simulink model "gm_db2_level5_final_hdlsss"  (R2021a)
settings: Solver=FixedStepDiscrete  StartTime=0.0  StopTime=0.2  RelTol=1e-3
libraries: hdlmdlgenlib x56
(part 2 of 4)

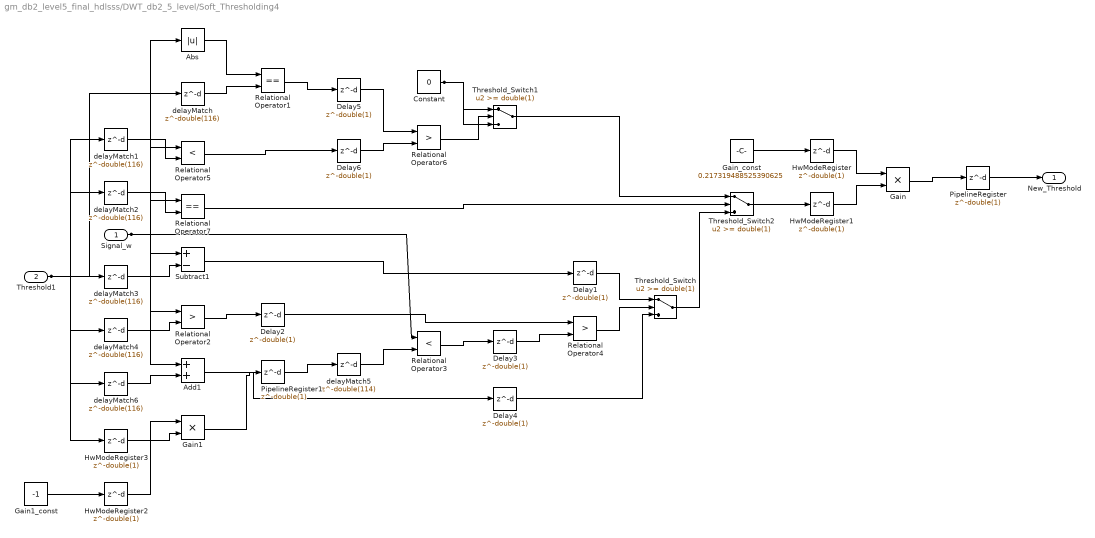
== system gm_db2_level5_final_hdlsss/DWT_db2_5_level/Soft_Thresholding4 ==
  Signal_w : Inport  OutDataTypeStr=fixdt(1, 16, 27)  PortDimensions=1  SampleTime=2.26757369614512e-05
  Threshold1 : Inport  Port=2  OutDataTypeStr=fixdt(0, 16, 27)  PortDimensions=1  SampleTime=2.26757369614512e-05
  Abs : Abs  SampleTime=2.26757369614512e-05  OutDataTypeStr=fixdt(0, 16, 28)
  Add1 : Sum  AccumDataTypeStr=fixdt(1, 16, 26)  OutDataTypeStr=fixdt(1, 16, 26)  SampleTime=2.26757369614512e-05
  Constant : Constant  Value=0  OutDataTypeStr=fixdt(1, 16, 4)  SampleTime=2.26757369614512e-05
  Delay{1..6} (6 alike) : Delay  DelayLength=double(1)  InitialCondition=0  SampleTime=2.26757369614512e-05
  Gain : Product  Inputs=**  OutDataTypeStr=fixdt(1, 16, 28)  SampleTime=2.26757369614512e-05
  Gain1 : Product  Inputs=**  OutDataTypeStr=fixdt(1, 16, 15)  SampleTime=2.26757369614512e-05
  Gain1_const : Constant  Value=-1  OutDataTypeStr=fixdt(1, 16, 15)  SampleTime=2.26757369614512e-05
  Gain_const : Constant  Value=0.217319488525390625  OutDataTypeStr=fixdt(0, 16, 18)  SampleTime=2.26757369614512e-05
  HwModeRegister{,1..3} (4 alike) : Delay  DelayLength=double(1)  InitialCondition=0  SampleTime=2.26757369614512e-05
  PipelineRegister : Delay  DelayLength=double(1)  InitialCondition=0  SampleTime=2.26757369614512e-05
  PipelineRegister1 : Delay  DelayLength=double(1)  InitialCondition=0  SampleTime=2.26757369614512e-05
  Relational Operator1 : RelationalOperator  Operator===  OutDataTypeStr=fixdt(1,16,0)  SampleTime=2.26757369614512e-05  RndMeth=Nearest
  Relational Operator2 : RelationalOperator  Operator=>  OutDataTypeStr=fixdt(1,16,0)  SampleTime=2.26757369614512e-05  RndMeth=Nearest
  Relational Operator3 : RelationalOperator  Operator=<  OutDataTypeStr=fixdt(1,16,0)  SampleTime=2.26757369614512e-05  RndMeth=Nearest
  Relational Operator4 : RelationalOperator  Operator=>  OutDataTypeStr=fixdt(1,16,0)  SampleTime=2.26757369614512e-05  RndMeth=Nearest
  Relational Operator5 : RelationalOperator  Operator=<  OutDataTypeStr=fixdt(1,16,0)  SampleTime=2.26757369614512e-05  RndMeth=Nearest
  Relational Operator6 : RelationalOperator  Operator=>  OutDataTypeStr=fixdt(1,16,0)  SampleTime=2.26757369614512e-05  RndMeth=Nearest
  Relational Operator7 : RelationalOperator  Operator===  OutDataTypeStr=fixdt(1,16,0)  SampleTime=2.26757369614512e-05  RndMeth=Nearest
  Subtract1 : Sum  Inputs=+-  AccumDataTypeStr=fixdt(1, 16, 25)  OutDataTypeStr=fixdt(1, 16, 25)  SampleTime=2.26757369614512e-05
  Threshold_Switch : Switch  Threshold=double(1)  OutDataTypeStr=fixdt(1, 16, 26)  SampleTime=2.26757369614512e-05
  Threshold_Switch1 : Switch  Threshold=double(1)  OutDataTypeStr=fixdt(1, 16, 4)  SampleTime=2.26757369614512e-05
  Threshold_Switch2 : Switch  Threshold=double(1)  OutDataTypeStr=fixdt(1, 16, 26)  SampleTime=2.26757369614512e-05
  delayMatch{,1..4,6} (6 alike) : Delay  DelayLength=double(116)  InitialCondition=0  SampleTime=2.26757369614512e-05
  delayMatch5 : Delay  DelayLength=double(114)  InitialCondition=0  SampleTime=2.26757369614512e-05
  New_Threshold : Outport  OutDataTypeStr=fixdt(1,16,28)  SampleTime=2.26757369614512e-05
  wires:
  delayMatch/1 -> Relational Operator1/2
  Abs/1 -> Relational Operator1/1
  Add1/1 -> Delay4/1
  Constant/1 -> Threshold_Switch1/3, Threshold_Switch1/1
  Delay1/1 -> Threshold_Switch/1
  Delay2/1 -> Relational Operator4/1
  Delay3/1 -> Relational Operator4/2
  Delay4/1 -> Threshold_Switch/3
  Delay5/1 -> Relational Operator6/1
  Delay6/1 -> Relational Operator6/2
  PipelineRegister/1 -> New_Threshold/1
  delayMatch5/1 -> Relational Operator3/2
  Relational Operator1/1 -> Delay5/1
  Relational Operator2/1 -> Delay2/1
  Relational Operator3/1 -> Delay3/1
  Relational Operator4/1 -> Threshold_Switch/2
  Relational Operator5/1 -> Delay6/1
  Relational Operator6/1 -> Threshold_Switch1/2
  Relational Operator7/1 -> Threshold_Switch2/2
  Subtract1/1 -> Delay1/1
  Threshold_Switch/1 -> Threshold_Switch2/3
  Threshold_Switch1/1 -> Threshold_Switch2/1
  Threshold_Switch2/1 -> HwModeRegister1/1
  Gain_const/1 -> HwModeRegister/1
  Gain1_const/1 -> HwModeRegister2/1
  Signal_w/1 -> Subtract1/1, Relational Operator7/1, Relational Operator5/1, Relational Operator3/1, Relational Operator2/1, Add1/1, Abs/1
  Threshold1/1 -> delayMatch6/1, delayMatch4/1, delayMatch3/1, delayMatch2/1, delayMatch1/1, delayMatch/1, HwModeRegister3/1
  delayMatch1/1 -> Relational Operator5/2
  delayMatch2/1 -> Relational Operator7/2
  delayMatch3/1 -> Subtract1/2
  delayMatch4/1 -> Relational Operator2/2
  delayMatch6/1 -> Add1/2
  PipelineRegister1/1 -> delayMatch5/1
  Gain/1 -> PipelineRegister/1
  HwModeRegister/1 -> Gain/1
  HwModeRegister1/1 -> Gain/2
  Gain1/1 -> PipelineRegister1/1
  HwModeRegister2/1 -> Gain1/1
  HwModeRegister3/1 -> Gain1/2

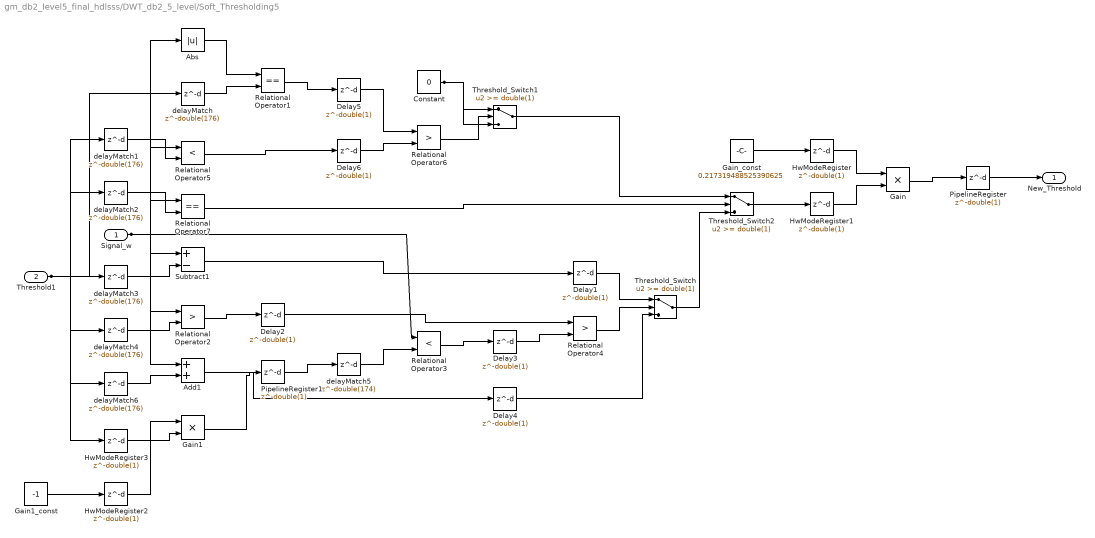
== system gm_db2_level5_final_hdlsss/DWT_db2_5_level/Soft_Thresholding5 ==
  Signal_w : Inport  OutDataTypeStr=fixdt(1, 16, 27)  PortDimensions=1  SampleTime=2.26757369614512e-05
  Threshold1 : Inport  Port=2  OutDataTypeStr=fixdt(0, 16, 27)  PortDimensions=1  SampleTime=2.26757369614512e-05
  Abs : Abs  SampleTime=2.26757369614512e-05  OutDataTypeStr=fixdt(0, 16, 28)
  Add1 : Sum  AccumDataTypeStr=fixdt(1, 16, 26)  OutDataTypeStr=fixdt(1, 16, 26)  SampleTime=2.26757369614512e-05
  Constant : Constant  Value=0  OutDataTypeStr=fixdt(1, 16, 4)  SampleTime=2.26757369614512e-05
  Delay{1..6} (6 alike) : Delay  DelayLength=double(1)  InitialCondition=0  SampleTime=2.26757369614512e-05
  Gain : Product  Inputs=**  OutDataTypeStr=fixdt(1, 16, 28)  SampleTime=2.26757369614512e-05
  Gain1 : Product  Inputs=**  OutDataTypeStr=fixdt(1, 16, 15)  SampleTime=2.26757369614512e-05
  Gain1_const : Constant  Value=-1  OutDataTypeStr=fixdt(1, 16, 15)  SampleTime=2.26757369614512e-05
  Gain_const : Constant  Value=0.217319488525390625  OutDataTypeStr=fixdt(0, 16, 18)  SampleTime=2.26757369614512e-05
  HwModeRegister{,1..3} (4 alike) : Delay  DelayLength=double(1)  InitialCondition=0  SampleTime=2.26757369614512e-05
  PipelineRegister : Delay  DelayLength=double(1)  InitialCondition=0  SampleTime=2.26757369614512e-05
  PipelineRegister1 : Delay  DelayLength=double(1)  InitialCondition=0  SampleTime=2.26757369614512e-05
  Relational Operator1 : RelationalOperator  Operator===  OutDataTypeStr=fixdt(1,16,0)  SampleTime=2.26757369614512e-05  RndMeth=Nearest
  Relational Operator2 : RelationalOperator  Operator=>  OutDataTypeStr=fixdt(1,16,0)  SampleTime=2.26757369614512e-05  RndMeth=Nearest
  Relational Operator3 : RelationalOperator  Operator=<  OutDataTypeStr=fixdt(1,16,0)  SampleTime=2.26757369614512e-05  RndMeth=Nearest
  Relational Operator4 : RelationalOperator  Operator=>  OutDataTypeStr=fixdt(1,16,0)  SampleTime=2.26757369614512e-05  RndMeth=Nearest
  Relational Operator5 : RelationalOperator  Operator=<  OutDataTypeStr=fixdt(1,16,0)  SampleTime=2.26757369614512e-05  RndMeth=Nearest
  Relational Operator6 : RelationalOperator  Operator=>  OutDataTypeStr=fixdt(1,16,0)  SampleTime=2.26757369614512e-05  RndMeth=Nearest
  Relational Operator7 : RelationalOperator  Operator===  OutDataTypeStr=fixdt(1,16,0)  SampleTime=2.26757369614512e-05  RndMeth=Nearest
  Subtract1 : Sum  Inputs=+-  AccumDataTypeStr=fixdt(1, 16, 25)  OutDataTypeStr=fixdt(1, 16, 25)  SampleTime=2.26757369614512e-05
  Threshold_Switch : Switch  Threshold=double(1)  OutDataTypeStr=fixdt(1, 16, 26)  SampleTime=2.26757369614512e-05
  Threshold_Switch1 : Switch  Threshold=double(1)  OutDataTypeStr=fixdt(1, 16, 4)  SampleTime=2.26757369614512e-05
  Threshold_Switch2 : Switch  Threshold=double(1)  OutDataTypeStr=fixdt(1, 16, 26)  SampleTime=2.26757369614512e-05
  delayMatch{,1..4,6} (6 alike) : Delay  DelayLength=double(176)  InitialCondition=0  SampleTime=2.26757369614512e-05
  delayMatch5 : Delay  DelayLength=double(174)  InitialCondition=0  SampleTime=2.26757369614512e-05
  New_Threshold : Outport  OutDataTypeStr=fixdt(1,16,28)  SampleTime=2.26757369614512e-05
  wires:
  delayMatch/1 -> Relational Operator1/2
  Abs/1 -> Relational Operator1/1
  Add1/1 -> Delay4/1
  Constant/1 -> Threshold_Switch1/3, Threshold_Switch1/1
  Delay1/1 -> Threshold_Switch/1
  Delay2/1 -> Relational Operator4/1
  Delay3/1 -> Relational Operator4/2
  Delay4/1 -> Threshold_Switch/3
  Delay5/1 -> Relational Operator6/1
  Delay6/1 -> Relational Operator6/2
  PipelineRegister/1 -> New_Threshold/1
  delayMatch5/1 -> Relational Operator3/2
  Relational Operator1/1 -> Delay5/1
  Relational Operator2/1 -> Delay2/1
  Relational Operator3/1 -> Delay3/1
  Relational Operator4/1 -> Threshold_Switch/2
  Relational Operator5/1 -> Delay6/1
  Relational Operator6/1 -> Threshold_Switch1/2
  Relational Operator7/1 -> Threshold_Switch2/2
  Subtract1/1 -> Delay1/1
  Threshold_Switch/1 -> Threshold_Switch2/3
  Threshold_Switch1/1 -> Threshold_Switch2/1
  Threshold_Switch2/1 -> HwModeRegister1/1
  Gain_const/1 -> HwModeRegister/1
  Gain1_const/1 -> HwModeRegister2/1
  Signal_w/1 -> Subtract1/1, Relational Operator7/1, Relational Operator5/1, Relational Operator3/1, Relational Operator2/1, Add1/1, Abs/1
  Threshold1/1 -> delayMatch6/1, delayMatch4/1, delayMatch3/1, delayMatch2/1, delayMatch1/1, delayMatch/1, HwModeRegister3/1
  delayMatch1/1 -> Relational Operator5/2
  delayMatch2/1 -> Relational Operator7/2
  delayMatch3/1 -> Subtract1/2
  delayMatch4/1 -> Relational Operator2/2
  delayMatch6/1 -> Add1/2
  PipelineRegister1/1 -> delayMatch5/1
  Gain/1 -> PipelineRegister/1
  HwModeRegister/1 -> Gain/1
  HwModeRegister1/1 -> Gain/2
  Gain1/1 -> PipelineRegister1/1
  HwModeRegister2/1 -> Gain1/1
  HwModeRegister3/1 -> Gain1/2

== system gm_db2_level5_final_hdlsss/DWT_db2_5_level/Threshold_Estimator ==
  Signal_w : Inport  OutDataTypeStr=fixdt(1, 16, 27)  PortDimensions=1  SampleTime=2.26757369614512e-05
  Absolute_Value : Subsystem
  HwModeRegister : Delay  DelayLength=double(1)  InitialCondition=0  SampleTime=2.26757369614512e-05
  HwModeRegister1 : Delay  DelayLength=double(1)  InitialCondition=0  SampleTime=2.26757369614512e-05
  Length : Constant  Value=2.30072021484375  OutDataTypeStr=fixdt(0, 16, 14)  SampleTime=2.26757369614512e-05
  Median : Subsystem
  Multiply : Product  Inputs=**  OutDataTypeStr=fixdt(0, 16, 27)  SampleTime=2.26757369614512e-05
  PipelineRegister : Delay  DelayLength=double(1)  InitialCondition=0  SampleTime=2.26757369614512e-05
  Threshold : Outport  OutDataTypeStr=fixdt(0,16,27)  SampleTime=2.26757369614512e-05  VectorParamsAs1DForOutWhenUnconnected=off
  wires:
  Absolute_Value/1(Out_Abs) -> Median/1(In_Abs)
  Length/1 -> HwModeRegister1/1
  Median/1(Median) -> HwModeRegister/1
  PipelineRegister/1 -> Threshold/1
  Signal_w/1 -> Absolute_Value/1(Signal_w)
  Multiply/1 -> PipelineRegister/1
  HwModeRegister/1 -> Multiply/1
  HwModeRegister1/1 -> Multiply/2

== system gm_db2_level5_final_hdlsss/DWT_db2_5_level/1st_Level_Decomp1/HiD_Even ==
  In_HiD_e : Inport  OutDataTypeStr=fixdt(0, 16, 23)  PortDimensions=1  SampleTime=2.26757369614512e-05
  Add : Sum  AccumDataTypeStr=fixdt(1, 16, 15)  OutDataTypeStr=fixdt(1, 16, 15)  SampleTime=2.26757369614512e-05
  Delay : Delay  DelayLength=double(1)  InitialCondition=0  SampleTime=2.26757369614512e-05
  HiD_0 : Constant  Value=-0.4829559326171875  OutDataTypeStr=fixdt(1, 16, 16)  SampleTime=2.26757369614512e-05
  HiD_2 : Constant  Value=-0.22414398193359375  OutDataTypeStr=fixdt(1, 16, 17)  SampleTime=2.26757369614512e-05
  HwModeRegister{,1..3} (4 alike) : Delay  DelayLength=double(1)  InitialCondition=0  SampleTime=2.26757369614512e-05
  Multiply : Product  Inputs=**  OutDataTypeStr=fixdt(1, 16, 15)  SampleTime=2.26757369614512e-05
  Multiply1 : Product  Inputs=**  OutDataTypeStr=fixdt(1, 16, 15)  SampleTime=2.26757369614512e-05
  PipelineRegister : Delay  DelayLength=double(1)  InitialCondition=0  SampleTime=2.26757369614512e-05
  PipelineRegister1 : Delay  DelayLength=double(1)  InitialCondition=0  SampleTime=2.26757369614512e-05
  Rate Transition : hdlmdlgenlib/Buffer
      settings: SourceProductBaseCode=SL
  delayMatch : Delay  DelayLength=double(1)  InitialCondition=0  SampleTime=2.26757369614512e-05
  Out_HiD_e : Outport  OutDataTypeStr=fixdt(1,16,15)  SampleTime=2.26757369614512e-05  VectorParamsAs1DForOutWhenUnconnected=off
  wires:
  Add/1 -> Out_HiD_e/1
  Delay/1 -> Rate Transition/1
  HiD_0/1 -> HwModeRegister/1
  HiD_2/1 -> HwModeRegister2/1
  PipelineRegister/1 -> Add/1
  delayMatch/1 -> Add/2
  Rate Transition/1 -> HwModeRegister3/1
  In_HiD_e/1 -> Delay/1, HwModeRegister1/1
  PipelineRegister1/1 -> delayMatch/1
  Multiply/1 -> PipelineRegister/1
  HwModeRegister/1 -> Multiply/1
  HwModeRegister1/1 -> Multiply/2
  Multiply1/1 -> PipelineRegister1/1
  HwModeRegister2/1 -> Multiply1/1
  HwModeRegister3/1 -> Multiply1/2

== system gm_db2_level5_final_hdlsss/DWT_db2_5_level/1st_Level_Decomp1/HiD_Odd ==
  In_HiD_o : Inport  OutDataTypeStr=fixdt(0, 16, 23)  PortDimensions=1  SampleTime=2.26757369614512e-05
  Add : Sum  AccumDataTypeStr=fixdt(1, 16, 22)  OutDataTypeStr=fixdt(0, 16, 24)  SampleTime=2.26757369614512e-05
  Delay : Delay  DelayLength=double(1)  InitialCondition=0  SampleTime=2.26757369614512e-05
  HiD_1 : Constant  Value=0.836517333984375  OutDataTypeStr=fixdt(0, 16, 16)  SampleTime=2.26757369614512e-05
  HiD_3 : Constant  Value=-0.1294097900390625  OutDataTypeStr=fixdt(1, 16, 17)  SampleTime=2.26757369614512e-05
  HwModeRegister{,1..3} (4 alike) : Delay  DelayLength=double(1)  InitialCondition=0  SampleTime=2.26757369614512e-05
  Multiply : Product  Inputs=**  OutDataTypeStr=fixdt(0, 16, 23)  SampleTime=2.26757369614512e-05
  Multiply1 : Product  Inputs=**  OutDataTypeStr=fixdt(1, 16, 15)  SampleTime=2.26757369614512e-05
  PipelineRegister : Delay  DelayLength=double(1)  InitialCondition=0  SampleTime=2.26757369614512e-05
  PipelineRegister1 : Delay  DelayLength=double(1)  InitialCondition=0  SampleTime=2.26757369614512e-05
  Rate Transition : hdlmdlgenlib/Buffer
      settings: SourceProductBaseCode=SL
  delayMatch : Delay  DelayLength=double(1)  InitialCondition=0  SampleTime=2.26757369614512e-05
  Out_HiD_o : Outport  OutDataTypeStr=fixdt(0,16,24)  SampleTime=2.26757369614512e-05  VectorParamsAs1DForOutWhenUnconnected=off
  wires:
  Add/1 -> Out_HiD_o/1
  Delay/1 -> Rate Transition/1
  HiD_1/1 -> HwModeRegister/1
  HiD_3/1 -> HwModeRegister2/1
  PipelineRegister/1 -> Add/1
  delayMatch/1 -> Add/2
  Rate Transition/1 -> HwModeRegister3/1
  In_HiD_o/1 -> Delay/1, HwModeRegister1/1
  PipelineRegister1/1 -> delayMatch/1
  Multiply/1 -> PipelineRegister/1
  HwModeRegister/1 -> Multiply/1
  HwModeRegister1/1 -> Multiply/2
  Multiply1/1 -> PipelineRegister1/1
  HwModeRegister2/1 -> Multiply1/1
  HwModeRegister3/1 -> Multiply1/2

== system gm_db2_level5_final_hdlsss/DWT_db2_5_level/1st_Level_Decomp1/LoD_Even ==
  In_LoD_e : Inport  OutDataTypeStr=fixdt(0, 16, 23)  PortDimensions=1  SampleTime=2.26757369614512e-05
  Add : Sum  AccumDataTypeStr=fixdt(1, 16, 22)  OutDataTypeStr=fixdt(1, 16, 23)  SampleTime=2.26757369614512e-05
  Delay : Delay  DelayLength=double(1)  InitialCondition=0  SampleTime=2.26757369614512e-05
  HwModeRegister{,1..3} (4 alike) : Delay  DelayLength=double(1)  InitialCondition=0  SampleTime=2.26757369614512e-05
  LoD_0 : Constant  Value=-0.1294097900390625  OutDataTypeStr=fixdt(1, 16, 17)  SampleTime=2.26757369614512e-05
  LoD_2 : Constant  Value=0.836517333984375  OutDataTypeStr=fixdt(0, 16, 16)  SampleTime=2.26757369614512e-05
  Multiply : Product  Inputs=**  OutDataTypeStr=fixdt(1, 16, 15)  SampleTime=2.26757369614512e-05
  Multiply1 : Product  Inputs=**  OutDataTypeStr=fixdt(0, 16, 23)  SampleTime=2.26757369614512e-05
  PipelineRegister : Delay  DelayLength=double(1)  InitialCondition=0  SampleTime=2.26757369614512e-05
  PipelineRegister1 : Delay  DelayLength=double(1)  InitialCondition=0  SampleTime=2.26757369614512e-05
  Rate Transition : hdlmdlgenlib/Buffer
      settings: SourceProductBaseCode=SL
  delayMatch : Delay  DelayLength=double(1)  InitialCondition=0  SampleTime=2.26757369614512e-05
  Out_LoD_e : Outport  OutDataTypeStr=fixdt(1,16,23)  SampleTime=2.26757369614512e-05  VectorParamsAs1DForOutWhenUnconnected=off
  wires:
  Add/1 -> Out_LoD_e/1
  Delay/1 -> Rate Transition/1
  LoD_0/1 -> HwModeRegister/1
  LoD_2/1 -> HwModeRegister2/1
  PipelineRegister/1 -> Add/1
  delayMatch/1 -> Add/2
  Rate Transition/1 -> HwModeRegister3/1
  In_LoD_e/1 -> Delay/1, HwModeRegister1/1
  PipelineRegister1/1 -> delayMatch/1
  Multiply/1 -> PipelineRegister/1
  HwModeRegister/1 -> Multiply/1
  HwModeRegister1/1 -> Multiply/2
  Multiply1/1 -> PipelineRegister1/1
  HwModeRegister2/1 -> Multiply1/1
  HwModeRegister3/1 -> Multiply1/2

== system gm_db2_level5_final_hdlsss/DWT_db2_5_level/1st_Level_Decomp1/LoD_Odd ==
  In_LoD_o : Inport  OutDataTypeStr=fixdt(0, 16, 23)  PortDimensions=1  SampleTime=2.26757369614512e-05
  Add : Sum  AccumDataTypeStr=fixdt(0, 16, 24)  OutDataTypeStr=fixdt(0, 16, 24)  SampleTime=2.26757369614512e-05
  Delay : Delay  DelayLength=double(1)  InitialCondition=0  SampleTime=2.26757369614512e-05
  HwModeRegister{,1..3} (4 alike) : Delay  DelayLength=double(1)  InitialCondition=0  SampleTime=2.26757369614512e-05
  LoD_1 : Constant  Value=0.22414398193359375  OutDataTypeStr=fixdt(0, 16, 18)  SampleTime=2.26757369614512e-05
  LoD_3 : Constant  Value=0.48296356201171875  OutDataTypeStr=fixdt(0, 16, 17)  SampleTime=2.26757369614512e-05
  Multiply : Product  Inputs=**  OutDataTypeStr=fixdt(0, 16, 25)  SampleTime=2.26757369614512e-05
  Multiply1 : Product  Inputs=**  OutDataTypeStr=fixdt(0, 16, 24)  SampleTime=2.26757369614512e-05
  PipelineRegister : Delay  DelayLength=double(1)  InitialCondition=0  SampleTime=2.26757369614512e-05
  PipelineRegister1 : Delay  DelayLength=double(1)  InitialCondition=0  SampleTime=2.26757369614512e-05
  Rate Transition : hdlmdlgenlib/Buffer
      settings: SourceProductBaseCode=SL
  delayMatch : Delay  DelayLength=double(1)  InitialCondition=0  SampleTime=2.26757369614512e-05
  Out_LoD_o : Outport  OutDataTypeStr=fixdt(0,16,24)  SampleTime=2.26757369614512e-05  VectorParamsAs1DForOutWhenUnconnected=off
  wires:
  Add/1 -> Out_LoD_o/1
  Delay/1 -> Rate Transition/1
  LoD_1/1 -> HwModeRegister/1
  LoD_3/1 -> HwModeRegister2/1
  PipelineRegister/1 -> Add/1
  delayMatch/1 -> Add/2
  Rate Transition/1 -> HwModeRegister3/1
  In_LoD_o/1 -> Delay/1, HwModeRegister1/1
  PipelineRegister1/1 -> delayMatch/1
  Multiply/1 -> PipelineRegister/1
  HwModeRegister/1 -> Multiply/1
  HwModeRegister1/1 -> Multiply/2
  Multiply1/1 -> PipelineRegister1/1
  HwModeRegister2/1 -> Multiply1/1
  HwModeRegister3/1 -> Multiply1/2

== system gm_db2_level5_final_hdlsss/DWT_db2_5_level/1st_Level_Decomp2/HiD_Even ==
  In_HiD_e : Inport  OutDataTypeStr=fixdt(1, 16, 22)  PortDimensions=1  SampleTime=2.26757369614512e-05
  Add : Sum  AccumDataTypeStr=fixdt(1, 16, 15)  OutDataTypeStr=fixdt(1, 16, 15)  SampleTime=2.26757369614512e-05
  Delay : Delay  DelayLength=double(1)  InitialCondition=0  SampleTime=2.26757369614512e-05
  HiD_0 : Constant  Value=-0.4829559326171875  OutDataTypeStr=fixdt(1, 16, 16)  SampleTime=2.26757369614512e-05
  HiD_2 : Constant  Value=-0.22414398193359375  OutDataTypeStr=fixdt(1, 16, 17)  SampleTime=2.26757369614512e-05
  HwModeRegister{,1..3} (4 alike) : Delay  DelayLength=double(1)  InitialCondition=0  SampleTime=2.26757369614512e-05
  Multiply : Product  Inputs=**  OutDataTypeStr=fixdt(1, 16, 15)  SampleTime=2.26757369614512e-05
  Multiply1 : Product  Inputs=**  OutDataTypeStr=fixdt(1, 16, 15)  SampleTime=2.26757369614512e-05
  PipelineRegister : Delay  DelayLength=double(1)  InitialCondition=0  SampleTime=2.26757369614512e-05
  PipelineRegister1 : Delay  DelayLength=double(1)  InitialCondition=0  SampleTime=2.26757369614512e-05
  Rate Transition : hdlmdlgenlib/Buffer
      settings: SourceProductBaseCode=SL
  delayMatch : Delay  DelayLength=double(1)  InitialCondition=0  SampleTime=2.26757369614512e-05
  Out_HiD_e : Outport  OutDataTypeStr=fixdt(1,16,15)  SampleTime=2.26757369614512e-05  VectorParamsAs1DForOutWhenUnconnected=off
  wires:
  Add/1 -> Out_HiD_e/1
  Delay/1 -> Rate Transition/1
  HiD_0/1 -> HwModeRegister/1
  HiD_2/1 -> HwModeRegister2/1
  PipelineRegister/1 -> Add/1
  delayMatch/1 -> Add/2
  Rate Transition/1 -> HwModeRegister3/1
  In_HiD_e/1 -> Delay/1, HwModeRegister1/1
  PipelineRegister1/1 -> delayMatch/1
  Multiply/1 -> PipelineRegister/1
  HwModeRegister/1 -> Multiply/1
  HwModeRegister1/1 -> Multiply/2
  Multiply1/1 -> PipelineRegister1/1
  HwModeRegister2/1 -> Multiply1/1
  HwModeRegister3/1 -> Multiply1/2

== system gm_db2_level5_final_hdlsss/DWT_db2_5_level/1st_Level_Decomp2/HiD_Odd ==
  In_HiD_o : Inport  OutDataTypeStr=fixdt(1, 16, 22)  PortDimensions=1  SampleTime=2.26757369614512e-05
  Add : Sum  AccumDataTypeStr=fixdt(1, 16, 23)  OutDataTypeStr=fixdt(0, 16, 24)  SampleTime=2.26757369614512e-05
  Delay : Delay  DelayLength=double(1)  InitialCondition=0  SampleTime=2.26757369614512e-05
  HiD_1 : Constant  Value=0.836517333984375  OutDataTypeStr=fixdt(0, 16, 16)  SampleTime=2.26757369614512e-05
  HiD_3 : Constant  Value=-0.1294097900390625  OutDataTypeStr=fixdt(1, 16, 17)  SampleTime=2.26757369614512e-05
  HwModeRegister{,1..3} (4 alike) : Delay  DelayLength=double(1)  InitialCondition=0  SampleTime=2.26757369614512e-05
  Multiply : Product  Inputs=**  OutDataTypeStr=fixdt(0, 16, 24)  SampleTime=2.26757369614512e-05
  Multiply1 : Product  Inputs=**  OutDataTypeStr=fixdt(1, 16, 15)  SampleTime=2.26757369614512e-05
  PipelineRegister : Delay  DelayLength=double(1)  InitialCondition=0  SampleTime=2.26757369614512e-05
  PipelineRegister1 : Delay  DelayLength=double(1)  InitialCondition=0  SampleTime=2.26757369614512e-05
  Rate Transition : hdlmdlgenlib/Buffer
      settings: SourceProductBaseCode=SL
  delayMatch : Delay  DelayLength=double(1)  InitialCondition=0  SampleTime=2.26757369614512e-05
  Out_HiD_o : Outport  OutDataTypeStr=fixdt(0,16,24)  SampleTime=2.26757369614512e-05  VectorParamsAs1DForOutWhenUnconnected=off
  wires:
  Add/1 -> Out_HiD_o/1
  Delay/1 -> Rate Transition/1
  HiD_1/1 -> HwModeRegister/1
  HiD_3/1 -> HwModeRegister2/1
  PipelineRegister/1 -> Add/1
  delayMatch/1 -> Add/2
  Rate Transition/1 -> HwModeRegister3/1
  In_HiD_o/1 -> Delay/1, HwModeRegister1/1
  PipelineRegister1/1 -> delayMatch/1
  Multiply/1 -> PipelineRegister/1
  HwModeRegister/1 -> Multiply/1
  HwModeRegister1/1 -> Multiply/2
  Multiply1/1 -> PipelineRegister1/1
  HwModeRegister2/1 -> Multiply1/1
  HwModeRegister3/1 -> Multiply1/2

== system gm_db2_level5_final_hdlsss/DWT_db2_5_level/1st_Level_Decomp2/LoD_Even ==
  In_LoD_e : Inport  OutDataTypeStr=fixdt(1, 16, 22)  PortDimensions=1  SampleTime=2.26757369614512e-05
  Add : Sum  AccumDataTypeStr=fixdt(1, 16, 23)  OutDataTypeStr=fixdt(1, 16, 23)  SampleTime=2.26757369614512e-05
  Delay : Delay  DelayLength=double(1)  InitialCondition=0  SampleTime=2.26757369614512e-05
  HwModeRegister{,1..3} (4 alike) : Delay  DelayLength=double(1)  InitialCondition=0  SampleTime=2.26757369614512e-05
  LoD_0 : Constant  Value=-0.1294097900390625  OutDataTypeStr=fixdt(1, 16, 17)  SampleTime=2.26757369614512e-05
  LoD_2 : Constant  Value=0.836517333984375  OutDataTypeStr=fixdt(0, 16, 16)  SampleTime=2.26757369614512e-05
  Multiply : Product  Inputs=**  OutDataTypeStr=fixdt(1, 16, 15)  SampleTime=2.26757369614512e-05
  Multiply1 : Product  Inputs=**  OutDataTypeStr=fixdt(0, 16, 24)  SampleTime=2.26757369614512e-05
  PipelineRegister : Delay  DelayLength=double(1)  InitialCondition=0  SampleTime=2.26757369614512e-05
  PipelineRegister1 : Delay  DelayLength=double(1)  InitialCondition=0  SampleTime=2.26757369614512e-05
  Rate Transition : hdlmdlgenlib/Buffer
      settings: SourceProductBaseCode=SL
  delayMatch : Delay  DelayLength=double(1)  InitialCondition=0  SampleTime=2.26757369614512e-05
  Out_LoD_e : Outport  OutDataTypeStr=fixdt(1,16,23)  SampleTime=2.26757369614512e-05  VectorParamsAs1DForOutWhenUnconnected=off
  wires:
  Add/1 -> Out_LoD_e/1
  Delay/1 -> Rate Transition/1
  LoD_0/1 -> HwModeRegister/1
  LoD_2/1 -> HwModeRegister2/1
  PipelineRegister/1 -> Add/1
  delayMatch/1 -> Add/2
  Rate Transition/1 -> HwModeRegister3/1
  In_LoD_e/1 -> Delay/1, HwModeRegister1/1
  PipelineRegister1/1 -> delayMatch/1
  Multiply/1 -> PipelineRegister/1
  HwModeRegister/1 -> Multiply/1
  HwModeRegister1/1 -> Multiply/2
  Multiply1/1 -> PipelineRegister1/1
  HwModeRegister2/1 -> Multiply1/1
  HwModeRegister3/1 -> Multiply1/2

== system gm_db2_level5_final_hdlsss/DWT_db2_5_level/1st_Level_Decomp2/LoD_Odd ==
  In_LoD_o : Inport  OutDataTypeStr=fixdt(1, 16, 22)  PortDimensions=1  SampleTime=2.26757369614512e-05
  Add : Sum  AccumDataTypeStr=fixdt(0, 16, 24)  OutDataTypeStr=fixdt(0, 16, 24)  SampleTime=2.26757369614512e-05
  Delay : Delay  DelayLength=double(1)  InitialCondition=0  SampleTime=2.26757369614512e-05
  HwModeRegister{,1..3} (4 alike) : Delay  DelayLength=double(1)  InitialCondition=0  SampleTime=2.26757369614512e-05
  LoD_1 : Constant  Value=0.22414398193359375  OutDataTypeStr=fixdt(0, 16, 18)  SampleTime=2.26757369614512e-05
  LoD_3 : Constant  Value=0.48296356201171875  OutDataTypeStr=fixdt(0, 16, 17)  SampleTime=2.26757369614512e-05
  Multiply : Product  Inputs=**  OutDataTypeStr=fixdt(0, 16, 26)  SampleTime=2.26757369614512e-05
  Multiply1 : Product  Inputs=**  OutDataTypeStr=fixdt(0, 16, 25)  SampleTime=2.26757369614512e-05
  PipelineRegister : Delay  DelayLength=double(1)  InitialCondition=0  SampleTime=2.26757369614512e-05
  PipelineRegister1 : Delay  DelayLength=double(1)  InitialCondition=0  SampleTime=2.26757369614512e-05
  Rate Transition : hdlmdlgenlib/Buffer
      settings: SourceProductBaseCode=SL
  delayMatch : Delay  DelayLength=double(1)  InitialCondition=0  SampleTime=2.26757369614512e-05
  Out_LoD_o : Outport  OutDataTypeStr=fixdt(0,16,24)  SampleTime=2.26757369614512e-05  VectorParamsAs1DForOutWhenUnconnected=off
  wires:
  Add/1 -> Out_LoD_o/1
  Delay/1 -> Rate Transition/1
  LoD_1/1 -> HwModeRegister/1
  LoD_3/1 -> HwModeRegister2/1
  PipelineRegister/1 -> Add/1
  delayMatch/1 -> Add/2
  Rate Transition/1 -> HwModeRegister3/1
  In_LoD_o/1 -> Delay/1, HwModeRegister1/1
  PipelineRegister1/1 -> delayMatch/1
  Multiply/1 -> PipelineRegister/1
  HwModeRegister/1 -> Multiply/1
  HwModeRegister1/1 -> Multiply/2
  Multiply1/1 -> PipelineRegister1/1
  HwModeRegister2/1 -> Multiply1/1
  HwModeRegister3/1 -> Multiply1/2

== system gm_db2_level5_final_hdlsss/DWT_db2_5_level/1st_Level_Decomp3/HiD_Even ==
  In_HiD_e : Inport  OutDataTypeStr=fixdt(0, 16, 24)  PortDimensions=1  SampleTime=2.26757369614512e-05
  Add : Sum  AccumDataTypeStr=fixdt(1, 16, 15)  OutDataTypeStr=fixdt(1, 16, 15)  SampleTime=2.26757369614512e-05
  Delay : Delay  DelayLength=double(1)  InitialCondition=0  SampleTime=2.26757369614512e-05
  HiD_0 : Constant  Value=-0.4829559326171875  OutDataTypeStr=fixdt(1, 16, 16)  SampleTime=2.26757369614512e-05
  HiD_2 : Constant  Value=-0.22414398193359375  OutDataTypeStr=fixdt(1, 16, 17)  SampleTime=2.26757369614512e-05
  HwModeRegister{,1..3} (4 alike) : Delay  DelayLength=double(1)  InitialCondition=0  SampleTime=2.26757369614512e-05
  Multiply : Product  Inputs=**  OutDataTypeStr=fixdt(1, 16, 15)  SampleTime=2.26757369614512e-05
  Multiply1 : Product  Inputs=**  OutDataTypeStr=fixdt(1, 16, 15)  SampleTime=2.26757369614512e-05
  PipelineRegister : Delay  DelayLength=double(1)  InitialCondition=0  SampleTime=2.26757369614512e-05
  PipelineRegister1 : Delay  DelayLength=double(1)  InitialCondition=0  SampleTime=2.26757369614512e-05
  Rate Transition : hdlmdlgenlib/Buffer
      settings: SourceProductBaseCode=SL
  delayMatch : Delay  DelayLength=double(1)  InitialCondition=0  SampleTime=2.26757369614512e-05
  Out_HiD_e : Outport  OutDataTypeStr=fixdt(1,16,15)  SampleTime=2.26757369614512e-05  VectorParamsAs1DForOutWhenUnconnected=off
  wires:
  Add/1 -> Out_HiD_e/1
  Delay/1 -> Rate Transition/1
  HiD_0/1 -> HwModeRegister/1
  HiD_2/1 -> HwModeRegister2/1
  PipelineRegister/1 -> Add/1
  delayMatch/1 -> Add/2
  Rate Transition/1 -> HwModeRegister3/1
  In_HiD_e/1 -> Delay/1, HwModeRegister1/1
  PipelineRegister1/1 -> delayMatch/1
  Multiply/1 -> PipelineRegister/1
  HwModeRegister/1 -> Multiply/1
  HwModeRegister1/1 -> Multiply/2
  Multiply1/1 -> PipelineRegister1/1
  HwModeRegister2/1 -> Multiply1/1
  HwModeRegister3/1 -> Multiply1/2

== system gm_db2_level5_final_hdlsss/DWT_db2_5_level/1st_Level_Decomp3/HiD_Odd ==
  In_HiD_o : Inport  OutDataTypeStr=fixdt(0, 16, 24)  PortDimensions=1  SampleTime=2.26757369614512e-05
  Add : Sum  AccumDataTypeStr=fixdt(1, 16, 23)  OutDataTypeStr=fixdt(0, 16, 24)  SampleTime=2.26757369614512e-05
  Delay : Delay  DelayLength=double(1)  InitialCondition=0  SampleTime=2.26757369614512e-05
  HiD_1 : Constant  Value=0.836517333984375  OutDataTypeStr=fixdt(0, 16, 16)  SampleTime=2.26757369614512e-05
  HiD_3 : Constant  Value=-0.1294097900390625  OutDataTypeStr=fixdt(1, 16, 17)  SampleTime=2.26757369614512e-05
  HwModeRegister{,1..3} (4 alike) : Delay  DelayLength=double(1)  InitialCondition=0  SampleTime=2.26757369614512e-05
  Multiply : Product  Inputs=**  OutDataTypeStr=fixdt(0, 16, 24)  SampleTime=2.26757369614512e-05
  Multiply1 : Product  Inputs=**  OutDataTypeStr=fixdt(1, 16, 15)  SampleTime=2.26757369614512e-05
  PipelineRegister : Delay  DelayLength=double(1)  InitialCondition=0  SampleTime=2.26757369614512e-05
  PipelineRegister1 : Delay  DelayLength=double(1)  InitialCondition=0  SampleTime=2.26757369614512e-05
  Rate Transition : hdlmdlgenlib/Buffer
      settings: SourceProductBaseCode=SL
  delayMatch : Delay  DelayLength=double(1)  InitialCondition=0  SampleTime=2.26757369614512e-05
  Out_HiD_o : Outport  OutDataTypeStr=fixdt(0,16,24)  SampleTime=2.26757369614512e-05  VectorParamsAs1DForOutWhenUnconnected=off
  wires:
  Add/1 -> Out_HiD_o/1
  Delay/1 -> Rate Transition/1
  HiD_1/1 -> HwModeRegister/1
  HiD_3/1 -> HwModeRegister2/1
  PipelineRegister/1 -> Add/1
  delayMatch/1 -> Add/2
  Rate Transition/1 -> HwModeRegister3/1
  In_HiD_o/1 -> Delay/1, HwModeRegister1/1
  PipelineRegister1/1 -> delayMatch/1
  Multiply/1 -> PipelineRegister/1
  HwModeRegister/1 -> Multiply/1
  HwModeRegister1/1 -> Multiply/2
  Multiply1/1 -> PipelineRegister1/1
  HwModeRegister2/1 -> Multiply1/1
  HwModeRegister3/1 -> Multiply1/2

== system gm_db2_level5_final_hdlsss/DWT_db2_5_level/1st_Level_Decomp3/LoD_Even ==
  In_LoD_e : Inport  OutDataTypeStr=fixdt(0, 16, 24)  PortDimensions=1  SampleTime=2.26757369614512e-05
  Add : Sum  AccumDataTypeStr=fixdt(1, 16, 23)  OutDataTypeStr=fixdt(1, 16, 23)  SampleTime=2.26757369614512e-05
  Delay : Delay  DelayLength=double(1)  InitialCondition=0  SampleTime=2.26757369614512e-05
  HwModeRegister{,1..3} (4 alike) : Delay  DelayLength=double(1)  InitialCondition=0  SampleTime=2.26757369614512e-05
  LoD_0 : Constant  Value=-0.1294097900390625  OutDataTypeStr=fixdt(1, 16, 17)  SampleTime=2.26757369614512e-05
  LoD_2 : Constant  Value=0.836517333984375  OutDataTypeStr=fixdt(0, 16, 16)  SampleTime=2.26757369614512e-05
  Multiply : Product  Inputs=**  OutDataTypeStr=fixdt(1, 16, 15)  SampleTime=2.26757369614512e-05
  Multiply1 : Product  Inputs=**  OutDataTypeStr=fixdt(0, 16, 24)  SampleTime=2.26757369614512e-05
  PipelineRegister : Delay  DelayLength=double(1)  InitialCondition=0  SampleTime=2.26757369614512e-05
  PipelineRegister1 : Delay  DelayLength=double(1)  InitialCondition=0  SampleTime=2.26757369614512e-05
  Rate Transition : hdlmdlgenlib/Buffer
      settings: SourceProductBaseCode=SL
  delayMatch : Delay  DelayLength=double(1)  InitialCondition=0  SampleTime=2.26757369614512e-05
  Out_LoD_e : Outport  OutDataTypeStr=fixdt(1,16,23)  SampleTime=2.26757369614512e-05  VectorParamsAs1DForOutWhenUnconnected=off
  wires:
  Add/1 -> Out_LoD_e/1
  Delay/1 -> Rate Transition/1
  LoD_0/1 -> HwModeRegister/1
  LoD_2/1 -> HwModeRegister2/1
  PipelineRegister/1 -> Add/1
  delayMatch/1 -> Add/2
  Rate Transition/1 -> HwModeRegister3/1
  In_LoD_e/1 -> Delay/1, HwModeRegister1/1
  PipelineRegister1/1 -> delayMatch/1
  Multiply/1 -> PipelineRegister/1
  HwModeRegister/1 -> Multiply/1
  HwModeRegister1/1 -> Multiply/2
  Multiply1/1 -> PipelineRegister1/1
  HwModeRegister2/1 -> Multiply1/1
  HwModeRegister3/1 -> Multiply1/2

== system gm_db2_level5_final_hdlsss/DWT_db2_5_level/1st_Level_Decomp3/LoD_Odd ==
  In_LoD_o : Inport  OutDataTypeStr=fixdt(0, 16, 24)  PortDimensions=1  SampleTime=2.26757369614512e-05
  Add : Sum  AccumDataTypeStr=fixdt(0, 16, 24)  OutDataTypeStr=fixdt(0, 16, 24)  SampleTime=2.26757369614512e-05
  Delay : Delay  DelayLength=double(1)  InitialCondition=0  SampleTime=2.26757369614512e-05
  HwModeRegister{,1..3} (4 alike) : Delay  DelayLength=double(1)  InitialCondition=0  SampleTime=2.26757369614512e-05
  LoD_1 : Constant  Value=0.22414398193359375  OutDataTypeStr=fixdt(0, 16, 18)  SampleTime=2.26757369614512e-05
  LoD_3 : Constant  Value=0.48296356201171875  OutDataTypeStr=fixdt(0, 16, 17)  SampleTime=2.26757369614512e-05
  Multiply : Product  Inputs=**  OutDataTypeStr=fixdt(0, 16, 26)  SampleTime=2.26757369614512e-05
  Multiply1 : Product  Inputs=**  OutDataTypeStr=fixdt(0, 16, 25)  SampleTime=2.26757369614512e-05
  PipelineRegister : Delay  DelayLength=double(1)  InitialCondition=0  SampleTime=2.26757369614512e-05
  PipelineRegister1 : Delay  DelayLength=double(1)  InitialCondition=0  SampleTime=2.26757369614512e-05
  Rate Transition : hdlmdlgenlib/Buffer
      settings: SourceProductBaseCode=SL
  delayMatch : Delay  DelayLength=double(1)  InitialCondition=0  SampleTime=2.26757369614512e-05
  Out_LoD_o : Outport  OutDataTypeStr=fixdt(0,16,24)  SampleTime=2.26757369614512e-05  VectorParamsAs1DForOutWhenUnconnected=off
  wires:
  Add/1 -> Out_LoD_o/1
  Delay/1 -> Rate Transition/1
  LoD_1/1 -> HwModeRegister/1
  LoD_3/1 -> HwModeRegister2/1
  PipelineRegister/1 -> Add/1
  delayMatch/1 -> Add/2
  Rate Transition/1 -> HwModeRegister3/1
  In_LoD_o/1 -> Delay/1, HwModeRegister1/1
  PipelineRegister1/1 -> delayMatch/1
  Multiply/1 -> PipelineRegister/1
  HwModeRegister/1 -> Multiply/1
  HwModeRegister1/1 -> Multiply/2
  Multiply1/1 -> PipelineRegister1/1
  HwModeRegister2/1 -> Multiply1/1
  HwModeRegister3/1 -> Multiply1/2

== system gm_db2_level5_final_hdlsss/DWT_db2_5_level/1st_Level_Decomp4/HiD_Even ==
  In_HiD_e : Inport  OutDataTypeStr=fixdt(0, 16, 24)  PortDimensions=1  SampleTime=2.26757369614512e-05
  Add : Sum  AccumDataTypeStr=fixdt(1, 16, 15)  OutDataTypeStr=fixdt(1, 16, 15)  SampleTime=2.26757369614512e-05
  Delay : Delay  DelayLength=double(1)  InitialCondition=0  SampleTime=2.26757369614512e-05
  HiD_0 : Constant  Value=-0.4829559326171875  OutDataTypeStr=fixdt(1, 16, 16)  SampleTime=2.26757369614512e-05
  HiD_2 : Constant  Value=-0.22414398193359375  OutDataTypeStr=fixdt(1, 16, 17)  SampleTime=2.26757369614512e-05
  HwModeRegister{,1..3} (4 alike) : Delay  DelayLength=double(1)  InitialCondition=0  SampleTime=2.26757369614512e-05
  Multiply : Product  Inputs=**  OutDataTypeStr=fixdt(1, 16, 15)  SampleTime=2.26757369614512e-05
  Multiply1 : Product  Inputs=**  OutDataTypeStr=fixdt(1, 16, 15)  SampleTime=2.26757369614512e-05
  PipelineRegister : Delay  DelayLength=double(1)  InitialCondition=0  SampleTime=2.26757369614512e-05
  PipelineRegister1 : Delay  DelayLength=double(1)  InitialCondition=0  SampleTime=2.26757369614512e-05
  Rate Transition : hdlmdlgenlib/Buffer
      settings: SourceProductBaseCode=SL
  delayMatch : Delay  DelayLength=double(1)  InitialCondition=0  SampleTime=2.26757369614512e-05
  Out_HiD_e : Outport  OutDataTypeStr=fixdt(1,16,15)  SampleTime=2.26757369614512e-05  VectorParamsAs1DForOutWhenUnconnected=off
  wires:
  Add/1 -> Out_HiD_e/1
  Delay/1 -> Rate Transition/1
  HiD_0/1 -> HwModeRegister/1
  HiD_2/1 -> HwModeRegister2/1
  PipelineRegister/1 -> Add/1
  delayMatch/1 -> Add/2
  Rate Transition/1 -> HwModeRegister3/1
  In_HiD_e/1 -> Delay/1, HwModeRegister1/1
  PipelineRegister1/1 -> delayMatch/1
  Multiply/1 -> PipelineRegister/1
  HwModeRegister/1 -> Multiply/1
  HwModeRegister1/1 -> Multiply/2
  Multiply1/1 -> PipelineRegister1/1
  HwModeRegister2/1 -> Multiply1/1
  HwModeRegister3/1 -> Multiply1/2

== system gm_db2_level5_final_hdlsss/DWT_db2_5_level/1st_Level_Decomp4/HiD_Odd ==
  In_HiD_o : Inport  OutDataTypeStr=fixdt(0, 16, 24)  PortDimensions=1  SampleTime=2.26757369614512e-05
  Add : Sum  AccumDataTypeStr=fixdt(1, 16, 23)  OutDataTypeStr=fixdt(0, 16, 24)  SampleTime=2.26757369614512e-05
  Delay : Delay  DelayLength=double(1)  InitialCondition=0  SampleTime=2.26757369614512e-05
  HiD_1 : Constant  Value=0.836517333984375  OutDataTypeStr=fixdt(0, 16, 16)  SampleTime=2.26757369614512e-05
  HiD_3 : Constant  Value=-0.1294097900390625  OutDataTypeStr=fixdt(1, 16, 17)  SampleTime=2.26757369614512e-05
  HwModeRegister{,1..3} (4 alike) : Delay  DelayLength=double(1)  InitialCondition=0  SampleTime=2.26757369614512e-05
  Multiply : Product  Inputs=**  OutDataTypeStr=fixdt(0, 16, 24)  SampleTime=2.26757369614512e-05
  Multiply1 : Product  Inputs=**  OutDataTypeStr=fixdt(1, 16, 15)  SampleTime=2.26757369614512e-05
  PipelineRegister : Delay  DelayLength=double(1)  InitialCondition=0  SampleTime=2.26757369614512e-05
  PipelineRegister1 : Delay  DelayLength=double(1)  InitialCondition=0  SampleTime=2.26757369614512e-05
  Rate Transition : hdlmdlgenlib/Buffer
      settings: SourceProductBaseCode=SL
  delayMatch : Delay  DelayLength=double(1)  InitialCondition=0  SampleTime=2.26757369614512e-05
  Out_HiD_o : Outport  OutDataTypeStr=fixdt(0,16,24)  SampleTime=2.26757369614512e-05  VectorParamsAs1DForOutWhenUnconnected=off
  wires:
  Add/1 -> Out_HiD_o/1
  Delay/1 -> Rate Transition/1
  HiD_1/1 -> HwModeRegister/1
  HiD_3/1 -> HwModeRegister2/1
  PipelineRegister/1 -> Add/1
  delayMatch/1 -> Add/2
  Rate Transition/1 -> HwModeRegister3/1
  In_HiD_o/1 -> Delay/1, HwModeRegister1/1
  PipelineRegister1/1 -> delayMatch/1
  Multiply/1 -> PipelineRegister/1
  HwModeRegister/1 -> Multiply/1
  HwModeRegister1/1 -> Multiply/2
  Multiply1/1 -> PipelineRegister1/1
  HwModeRegister2/1 -> Multiply1/1
  HwModeRegister3/1 -> Multiply1/2

== system gm_db2_level5_final_hdlsss/DWT_db2_5_level/1st_Level_Decomp4/LoD_Even ==
  In_LoD_e : Inport  OutDataTypeStr=fixdt(0, 16, 24)  PortDimensions=1  SampleTime=2.26757369614512e-05
  Add : Sum  AccumDataTypeStr=fixdt(1, 16, 23)  OutDataTypeStr=fixdt(1, 16, 23)  SampleTime=2.26757369614512e-05
  Delay : Delay  DelayLength=double(1)  InitialCondition=0  SampleTime=2.26757369614512e-05
  HwModeRegister{,1..3} (4 alike) : Delay  DelayLength=double(1)  InitialCondition=0  SampleTime=2.26757369614512e-05
  LoD_0 : Constant  Value=-0.1294097900390625  OutDataTypeStr=fixdt(1, 16, 17)  SampleTime=2.26757369614512e-05
  LoD_2 : Constant  Value=0.836517333984375  OutDataTypeStr=fixdt(0, 16, 16)  SampleTime=2.26757369614512e-05
  Multiply : Product  Inputs=**  OutDataTypeStr=fixdt(1, 16, 15)  SampleTime=2.26757369614512e-05
  Multiply1 : Product  Inputs=**  OutDataTypeStr=fixdt(0, 16, 24)  SampleTime=2.26757369614512e-05
  PipelineRegister : Delay  DelayLength=double(1)  InitialCondition=0  SampleTime=2.26757369614512e-05
  PipelineRegister1 : Delay  DelayLength=double(1)  InitialCondition=0  SampleTime=2.26757369614512e-05
  Rate Transition : hdlmdlgenlib/Buffer
      settings: SourceProductBaseCode=SL
  delayMatch : Delay  DelayLength=double(1)  InitialCondition=0  SampleTime=2.26757369614512e-05
  Out_LoD_e : Outport  OutDataTypeStr=fixdt(1,16,23)  SampleTime=2.26757369614512e-05  VectorParamsAs1DForOutWhenUnconnected=off
  wires:
  Add/1 -> Out_LoD_e/1
  Delay/1 -> Rate Transition/1
  LoD_0/1 -> HwModeRegister/1
  LoD_2/1 -> HwModeRegister2/1
  PipelineRegister/1 -> Add/1
  delayMatch/1 -> Add/2
  Rate Transition/1 -> HwModeRegister3/1
  In_LoD_e/1 -> Delay/1, HwModeRegister1/1
  PipelineRegister1/1 -> delayMatch/1
  Multiply/1 -> PipelineRegister/1
  HwModeRegister/1 -> Multiply/1
  HwModeRegister1/1 -> Multiply/2
  Multiply1/1 -> PipelineRegister1/1
  HwModeRegister2/1 -> Multiply1/1
  HwModeRegister3/1 -> Multiply1/2

== system gm_db2_level5_final_hdlsss/DWT_db2_5_level/1st_Level_Decomp4/LoD_Odd ==
  In_LoD_o : Inport  OutDataTypeStr=fixdt(0, 16, 24)  PortDimensions=1  SampleTime=2.26757369614512e-05
  Add : Sum  AccumDataTypeStr=fixdt(0, 16, 24)  OutDataTypeStr=fixdt(0, 16, 24)  SampleTime=2.26757369614512e-05
  Delay : Delay  DelayLength=double(1)  InitialCondition=0  SampleTime=2.26757369614512e-05
  HwModeRegister{,1..3} (4 alike) : Delay  DelayLength=double(1)  InitialCondition=0  SampleTime=2.26757369614512e-05
  LoD_1 : Constant  Value=0.22414398193359375  OutDataTypeStr=fixdt(0, 16, 18)  SampleTime=2.26757369614512e-05
  LoD_3 : Constant  Value=0.48296356201171875  OutDataTypeStr=fixdt(0, 16, 17)  SampleTime=2.26757369614512e-05
  Multiply : Product  Inputs=**  OutDataTypeStr=fixdt(0, 16, 26)  SampleTime=2.26757369614512e-05
  Multiply1 : Product  Inputs=**  OutDataTypeStr=fixdt(0, 16, 25)  SampleTime=2.26757369614512e-05
  PipelineRegister : Delay  DelayLength=double(1)  InitialCondition=0  SampleTime=2.26757369614512e-05
  PipelineRegister1 : Delay  DelayLength=double(1)  InitialCondition=0  SampleTime=2.26757369614512e-05
  Rate Transition : hdlmdlgenlib/Buffer
      settings: SourceProductBaseCode=SL
  delayMatch : Delay  DelayLength=double(1)  InitialCondition=0  SampleTime=2.26757369614512e-05
  Out_LoD_o : Outport  OutDataTypeStr=fixdt(0,16,24)  SampleTime=2.26757369614512e-05  VectorParamsAs1DForOutWhenUnconnected=off
  wires:
  Add/1 -> Out_LoD_o/1
  Delay/1 -> Rate Transition/1
  LoD_1/1 -> HwModeRegister/1
  LoD_3/1 -> HwModeRegister2/1
  PipelineRegister/1 -> Add/1
  delayMatch/1 -> Add/2
  Rate Transition/1 -> HwModeRegister3/1
  In_LoD_o/1 -> Delay/1, HwModeRegister1/1
  PipelineRegister1/1 -> delayMatch/1
  Multiply/1 -> PipelineRegister/1
  HwModeRegister/1 -> Multiply/1
  HwModeRegister1/1 -> Multiply/2
  Multiply1/1 -> PipelineRegister1/1
  HwModeRegister2/1 -> Multiply1/1
  HwModeRegister3/1 -> Multiply1/2

== system gm_db2_level5_final_hdlsss/DWT_db2_5_level/1st_Level_Decomp5/HiD_Even ==
  In_HiD_e : Inport  OutDataTypeStr=fixdt(0, 16, 24)  PortDimensions=1  SampleTime=2.26757369614512e-05
  Add : Sum  AccumDataTypeStr=fixdt(1, 16, 15)  OutDataTypeStr=fixdt(1, 16, 15)  SampleTime=2.26757369614512e-05
  Delay : Delay  DelayLength=double(1)  InitialCondition=0  SampleTime=2.26757369614512e-05
  HiD_0 : Constant  Value=-0.4829559326171875  OutDataTypeStr=fixdt(1, 16, 16)  SampleTime=2.26757369614512e-05
  HiD_2 : Constant  Value=-0.22414398193359375  OutDataTypeStr=fixdt(1, 16, 17)  SampleTime=2.26757369614512e-05
  HwModeRegister{,1..3} (4 alike) : Delay  DelayLength=double(1)  InitialCondition=0  SampleTime=2.26757369614512e-05
  Multiply : Product  Inputs=**  OutDataTypeStr=fixdt(1, 16, 15)  SampleTime=2.26757369614512e-05
  Multiply1 : Product  Inputs=**  OutDataTypeStr=fixdt(1, 16, 15)  SampleTime=2.26757369614512e-05
  PipelineRegister : Delay  DelayLength=double(1)  InitialCondition=0  SampleTime=2.26757369614512e-05
  PipelineRegister1 : Delay  DelayLength=double(1)  InitialCondition=0  SampleTime=2.26757369614512e-05
  Rate Transition : hdlmdlgenlib/Buffer
      settings: SourceProductBaseCode=SL
  delayMatch : Delay  DelayLength=double(1)  InitialCondition=0  SampleTime=2.26757369614512e-05
  Out_HiD_e : Outport  OutDataTypeStr=fixdt(1,16,15)  SampleTime=2.26757369614512e-05  VectorParamsAs1DForOutWhenUnconnected=off
  wires:
  Add/1 -> Out_HiD_e/1
  Delay/1 -> Rate Transition/1
  HiD_0/1 -> HwModeRegister/1
  HiD_2/1 -> HwModeRegister2/1
  PipelineRegister/1 -> Add/1
  delayMatch/1 -> Add/2
  Rate Transition/1 -> HwModeRegister3/1
  In_HiD_e/1 -> Delay/1, HwModeRegister1/1
  PipelineRegister1/1 -> delayMatch/1
  Multiply/1 -> PipelineRegister/1
  HwModeRegister/1 -> Multiply/1
  HwModeRegister1/1 -> Multiply/2
  Multiply1/1 -> PipelineRegister1/1
  HwModeRegister2/1 -> Multiply1/1
  HwModeRegister3/1 -> Multiply1/2

== system gm_db2_level5_final_hdlsss/DWT_db2_5_level/1st_Level_Decomp5/HiD_Odd ==
  In_HiD_o : Inport  OutDataTypeStr=fixdt(0, 16, 24)  PortDimensions=1  SampleTime=2.26757369614512e-05
  Add : Sum  AccumDataTypeStr=fixdt(1, 16, 23)  OutDataTypeStr=fixdt(0, 16, 25)  SampleTime=2.26757369614512e-05
  Delay : Delay  DelayLength=double(1)  InitialCondition=0  SampleTime=2.26757369614512e-05
  HiD_1 : Constant  Value=0.836517333984375  OutDataTypeStr=fixdt(0, 16, 16)  SampleTime=2.26757369614512e-05
  HiD_3 : Constant  Value=-0.1294097900390625  OutDataTypeStr=fixdt(1, 16, 17)  SampleTime=2.26757369614512e-05
  HwModeRegister{,1..3} (4 alike) : Delay  DelayLength=double(1)  InitialCondition=0  SampleTime=2.26757369614512e-05
  Multiply : Product  Inputs=**  OutDataTypeStr=fixdt(0, 16, 24)  SampleTime=2.26757369614512e-05
  Multiply1 : Product  Inputs=**  OutDataTypeStr=fixdt(1, 16, 15)  SampleTime=2.26757369614512e-05
  PipelineRegister : Delay  DelayLength=double(1)  InitialCondition=0  SampleTime=2.26757369614512e-05
  PipelineRegister1 : Delay  DelayLength=double(1)  InitialCondition=0  SampleTime=2.26757369614512e-05
  Rate Transition : hdlmdlgenlib/Buffer
      settings: SourceProductBaseCode=SL
  delayMatch : Delay  DelayLength=double(1)  InitialCondition=0  SampleTime=2.26757369614512e-05
  Out_HiD_o : Outport  OutDataTypeStr=fixdt(0,16,25)  SampleTime=2.26757369614512e-05  VectorParamsAs1DForOutWhenUnconnected=off
  wires:
  Add/1 -> Out_HiD_o/1
  Delay/1 -> Rate Transition/1
  HiD_1/1 -> HwModeRegister/1
  HiD_3/1 -> HwModeRegister2/1
  PipelineRegister/1 -> Add/1
  delayMatch/1 -> Add/2
  Rate Transition/1 -> HwModeRegister3/1
  In_HiD_o/1 -> Delay/1, HwModeRegister1/1
  PipelineRegister1/1 -> delayMatch/1
  Multiply/1 -> PipelineRegister/1
  HwModeRegister/1 -> Multiply/1
  HwModeRegister1/1 -> Multiply/2
  Multiply1/1 -> PipelineRegister1/1
  HwModeRegister2/1 -> Multiply1/1
  HwModeRegister3/1 -> Multiply1/2

== system gm_db2_level5_final_hdlsss/DWT_db2_5_level/1st_Level_Decomp5/LoD_Even ==
  In_LoD_e : Inport  OutDataTypeStr=fixdt(0, 16, 24)  PortDimensions=1  SampleTime=2.26757369614512e-05
  Add : Sum  AccumDataTypeStr=fixdt(1, 16, 23)  OutDataTypeStr=fixdt(1, 16, 24)  SampleTime=2.26757369614512e-05
  Delay : Delay  DelayLength=double(1)  InitialCondition=0  SampleTime=2.26757369614512e-05
  HwModeRegister{,1..3} (4 alike) : Delay  DelayLength=double(1)  InitialCondition=0  SampleTime=2.26757369614512e-05
  LoD_0 : Constant  Value=-0.1294097900390625  OutDataTypeStr=fixdt(1, 16, 17)  SampleTime=2.26757369614512e-05
  LoD_2 : Constant  Value=0.836517333984375  OutDataTypeStr=fixdt(0, 16, 16)  SampleTime=2.26757369614512e-05
  Multiply : Product  Inputs=**  OutDataTypeStr=fixdt(1, 16, 15)  SampleTime=2.26757369614512e-05
  Multiply1 : Product  Inputs=**  OutDataTypeStr=fixdt(0, 16, 24)  SampleTime=2.26757369614512e-05
  PipelineRegister : Delay  DelayLength=double(1)  InitialCondition=0  SampleTime=2.26757369614512e-05
  PipelineRegister1 : Delay  DelayLength=double(1)  InitialCondition=0  SampleTime=2.26757369614512e-05
  Rate Transition : hdlmdlgenlib/Buffer
      settings: SourceProductBaseCode=SL
  delayMatch : Delay  DelayLength=double(1)  InitialCondition=0  SampleTime=2.26757369614512e-05
  Out_LoD_e : Outport  OutDataTypeStr=fixdt(1,16,24)  SampleTime=2.26757369614512e-05  VectorParamsAs1DForOutWhenUnconnected=off
  wires:
  Add/1 -> Out_LoD_e/1
  Delay/1 -> Rate Transition/1
  LoD_0/1 -> HwModeRegister/1
  LoD_2/1 -> HwModeRegister2/1
  PipelineRegister/1 -> Add/1
  delayMatch/1 -> Add/2
  Rate Transition/1 -> HwModeRegister3/1
  In_LoD_e/1 -> Delay/1, HwModeRegister1/1
  PipelineRegister1/1 -> delayMatch/1
  Multiply/1 -> PipelineRegister/1
  HwModeRegister/1 -> Multiply/1
  HwModeRegister1/1 -> Multiply/2
  Multiply1/1 -> PipelineRegister1/1
  HwModeRegister2/1 -> Multiply1/1
  HwModeRegister3/1 -> Multiply1/2
